simulink model "sl_groundvehicleDynamicsKalman"  (R2025a)
settings: Solver=VariableStepAuto  StartTime=0.0  StopTime=200  FixedStep=0.01  RelTol=1e-5  EnableMultiTasking=on
InitFcn:
  | mdl_robot;
values from neighbouring files (symbols this model uses):
  optimized_waypoints = two_opt_nn_multi_optimisation(cuztomized_wp)    [mdl_robot.m]
undefined symbols (not defined in the file or in its folder): Discrete, robot, Time
libraries: simulink x8, mobileRoboticsLib x5, simulink_extras x2, ctrlSharedLib x1, sharedTrackingLibrary x1
settings Model: Creator=sriramn  LastModifiedBy=login
settings SolverCC: ZeroCrossAlgorithm=Adaptive  AlgebraicLoopSolver=TrustRegion
settings DataIOCC: LimitDataPoints=on  SaveFormat=Array  ReturnWorkspaceOutputs=off
settings OptimizationCC: ReuseModelBlockBuffer=off  LifeSpan=inf
settings DebuggingCC: SolverPrmCheckMsg=warning  UnconnectedInputMsg=warning  UnconnectedOutputMsg=warning  UnconnectedLineMsg=warning  AllowSymbolicDim=off  SFUnexpectedBacktrackingDiag=warning  SFNoUnconditionalDefaultTransitionDiag=warning  SFExecutionAtInitializationDiag=none  ArithmeticOperatorsInVariantConditions=warning
settings HardwareCC: ProdBitPerPointer=32.0  ProdBitPerSizeT=32.0  ProdBitPerPtrDiffT=32.0  ProdLargestAtomicFloat=None  ProdIntDivRoundTo=Undefined  ProdEndianess=Unspecified  ProdWordSize=32.0  ProdHWDeviceType=32-bit Generic
settings ModelReferenceCC: EnableRefExpFcnMdlSchedulingChecks=on  ModelReferenceMinAlgLoopOccurrences=on  PropagateSignalLabelsOutOfModel=off
settings SFSimCC: SimUseLocalCustomCode=off  CustomCodeUndefinedFunction=UseInterfaceOnly
settings RTWCC: RTWUseLocalCustomCode=off  GPUComputeCapability=3.5
settings CodeAppCC: StateflowObjectComments=on
settings GRTTargetCC: TargetLangStandard=C89/C90 (ANSI)
settings ConfigComp: CovMetricSettings=dw  CovSaveCumulativeToWorkspaceVar=on  CovSaveSingleToWorkspaceVar=on  CovExternalEMLEnable=off  CovSFcnEnable=off
settings SimscapeCC: SimscapeLogDataHistory=5000  SimscapeLogDecimation=1  SimscapeNormalizeSystem=off
settings ConfigurationSet: Description=SimMechanics 2G
settings ExplorerConfigSet: InternalSimMechanicsExplorerSettings="<ExplorerConfiguration><canonicalview>planar_xy</canonicalview><AnimationSetting><BasePlaybackSpeed>1.0</BasePlaybackSpeed><PlaybackSpeedFactor>1.0</PlaybackSpeedFactor></AnimationSetting><TilePanel><TileInfo><Tiles Columns=\"1\" Count=\"1\" Rows=\"1\"><Column Left=\"2\" Weight=\"1\"/><Column Left=\"1628\"/><Row Top=\"2\" Weight=\"1\"/><Row Top=\"1072\"/><Tile Height=\"1\" Width=\"1\" X=\"0\" Y=\"0\"/></Tiles></TileInfo><SceneInfo><SceneViewer><BGColor><R>0.60000002384185791</R><G>0.60000002384185791</G><B>0.60000002384185791</B></BGColor><Camera><Position><X>0.22951840878551699</X><Y>0.32651610611526627</Y><Z>-0.27215421354393321</Z></Position><Center><X>-0.15775714411666431</X><Y>-0.15462825985839526</Y><Z>0.065702552916005602</Z></Center><Up><X>-0.56030137557930915</X><Y>0.72817587161684794</Y><Z>0.39474329445726858</Z></Up><Left>-0.21481383955700509</Left><Right>0.21481383955700509</Right><Bottom>-0.27569784609469139</Bottom><Top>0.27569784609469139</Top></Camera></SceneViewer></SceneInfo></TilePanel></ExplorerConfiguration>"

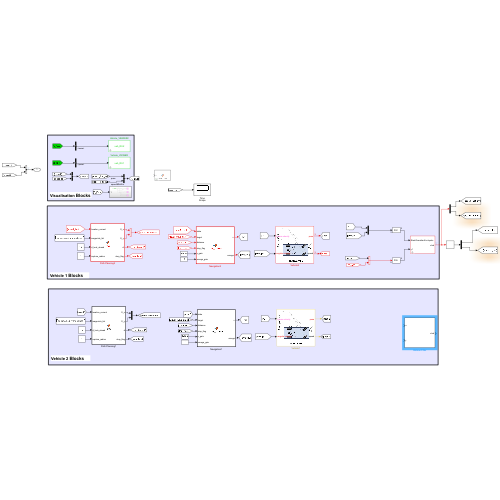
[thumbnail: Simulink's stored preview of the top-level diagram]
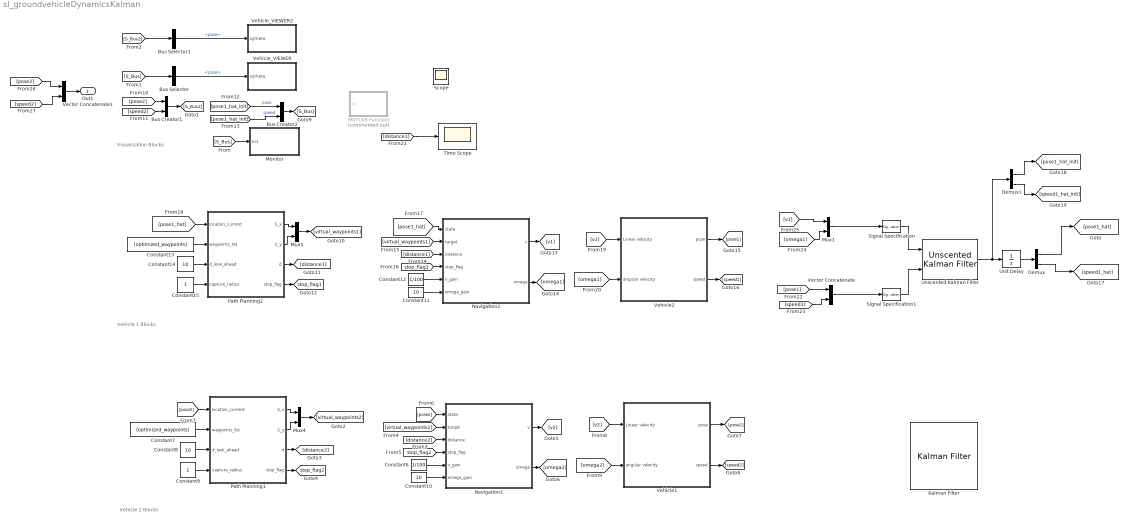
== system sl_groundvehicleDynamicsKalman ==
  note: Visualisation Blocks
  note: Vehicle 1 Blocks
  note: Vehicle 2 Blocks
  Bus Creator1 : BusCreator  Inputs=2
  Bus Creator2 : BusCreator  Inputs=2
  Bus Selector : BusSelector  OutputSignals=pose
  Bus Selector1 : BusSelector  OutputSignals=pose
  Constant{8,10..11,14} (4 alike) : Constant  Value=10
  Constant12 : Constant  Value=1/100
  Constant13 : Constant  Value=[optimized_waypoints]
  Constant15 : Constant
  Constant6 : Constant  Value=1/100
  Constant7 : Constant  Value=[optimized_waypoints]
  Constant9 : Constant
  Demux : Demux  Outputs=2
  Demux1 : Demux  Outputs=2
  Kalman Filter : ctrlSharedLib/Kalman Filter  TimeDomain=Discrete-Time  UseCurrentEstimator=on  ModelSource=LTI State-Space Variable  ModelSourceVariable=ss(0.95,1,1,0,1)  A=0.95  B=1  C=1  D=0  NumberOfStates=1  NumberOfInputs=1  NumberOfOutputs=1  InitialEstimateSource=Dialog  X0=0  P0=10  UseK=off  UseGH=off  NumberOfProcessNoiseInputs=1  G=1  TimeInvariantG=on  H=0  TimeInvariantH=on  Q=0.05  TimeInvariantQ=on  R=1  TimeInvariantR=on  N=0  TimeInvariantN=on  AddInputPort=on  AddEnablePort=off  OutputEstimatedY=off  OutputP=off  Ts=-1
  MATLAB Function : MATLAB Function  Commented=on  TreatAsAtomicUnit=on
  Monitor : Subsystem
  Mux1 : Mux  Inputs=2
  Mux4 : Mux  Inputs=2
  Mux5 : Mux  Inputs=2
  Navigation1 : MATLAB Function  TreatAsAtomicUnit=on
  Navigation2 : MATLAB Function  TreatAsAtomicUnit=on
  Path Planning1 : MATLAB Function  TreatAsAtomicUnit=on
  Path Planning2 : MATLAB Function  TreatAsAtomicUnit=on
  Signal Specification : SignalSpecification  Dimensions=2
  Signal Specification1 : SignalSpecification  Dimensions=6
  Time Scope : Scope
      settings: TimeUnits=Metric (based on Time Span)  ActiveDisplayYMinimum=-32041.582184274124  ActiveDisplayYMaximum=45911.6958514482  YLabel=Amplitude  DataLoggingVariableName=ScopeData3
  Unit Delay : UnitDelay  InitialCondition=[0;0;0;0;0;0]  SampleTime=-1  HasFrameUpgradeWarning=on
  Unscented Kalman Filter : sharedTrackingLibrary/Unscented Kalman Filter  StateTransitionFcn=fState  HasAdditiveProcessNoise=Additive  ProcessNoise=Q  HasTimeVaryingProcessNoise=off  HasStateTransitionFcnExtraArgument=1  InitialState=initial_state  InitialStateCovariance=P0  Alpha=1e-3  Beta=2  Kappa=0  MeasurementFcn1=hMeas  HasMeasurementEnablePort1=off  HasAdditiveMeasurementNoise1=Additive  MeasurementNoise1=R  HasTimeVaryingMeasurementNoise1=off  HasMeasurementFcnExtraArgument1=0  HasMeasurementWrapping1=on  MeasurementFcn2=myMeasurementFcn  HasMeasurementEnablePort2=off  HasAdditiveMeasurementNoise2=Additive  MeasurementNoise2=1  HasTimeVaryingMeasurementNoise2=off  HasMeasurementFcnExtraArgument2=0  HasMeasurementWrapping2=off  MeasurementFcn3=myMeasurementFcn  HasMeasurementEnablePort3=off  HasAdditiveMeasurementNoise3=Additive  MeasurementNoise3=1  HasTimeVaryingMeasurementNoise3=off  HasMeasurementFcnExtraArgument3=0  HasMeasurementWrapping3=off  MeasurementFcn4=myMeasurementFcn  HasMeasurementEnablePort4=off  HasAdditiveMeasurementNoise4=Additive  MeasurementNoise4=1  HasTimeVaryingMeasurementNoise4=off  HasMeasurementFcnExtraArgument4=0  HasMeasurementWrapping4=off  MeasurementFcn5=myMeasurementFcn  HasMeasurementEnablePort5=off  HasAdditiveMeasurementNoise5=Additive  MeasurementNoise5=1  HasTimeVaryingMeasurementNoise5=off  HasMeasurementFcnExtraArgument5=0  HasMeasurementWrapping5=off  EnableMultirate=off  StateTransitionFcnSampleTime=1  MeasurementFcn1SampleTime=1  MeasurementFcn2SampleTime=1  MeasurementFcn3SampleTime=1  MeasurementFcn4SampleTime=1  MeasurementFcn5SampleTime=1  UseCurrentEstimator=on  OutputStateCovariance=off  DataType=double  SampleTime=0.05  NumberOfMeasurements=1
      settings: LibrarySourceBlock=cstblocks/State Estimation/Unscented Kalman Filter
  Vector Concatenate : Concatenate
  Vector Concatenate1 : Concatenate
  Vehicle1 : Subsystem
      mask Display: image('vehicle.jpg');
  Vehicle2 : Subsystem
      mask Display: image('vehicle.jpg');
  Vehicle_VIEWER : Subsystem  mask{wp_mat=optimized_waypoints, veh_ID_num=1, veh_init_xytheta=[robot.X robot.Y robot.Theta], Ts=0.05}
      mask prompts: wp_mat "Waypoint matrix for arena [x_col, y_col] (m)"; veh_ID_num "Vehicle ID number"; veh_init_xytheta "Initial pose [x,y,theta]"; Ts "Sample time for updating animation (secs)"
      mask TypeOptions veh_ID_num: 1 | 2 | 3 | 4
      mask DialogControl Control2 Prompt: Animate simulation of Differential Drive Robot (DDR)
      mask Display: fprintf('veh_ID=%d',veh_ID_num);
  Vehicle_VIEWER2 : Subsystem  mask{wp_mat=optimized_waypoints, veh_ID_num=2, veh_init_xytheta=[robot.X robot.Y robot.Theta], Ts=0.05}
      mask prompts: wp_mat "Waypoint matrix for arena [x_col, y_col] (m)"; veh_ID_num "Vehicle ID number"; veh_init_xytheta "Initial pose [x,y,theta]"; Ts "Sample time for updating animation (secs)"
      mask TypeOptions veh_ID_num: 1 | 2 | 3 | 4
      mask DialogControl Control2 Prompt: Animate simulation of Differential Drive Robot (DDR)
      mask Display: fprintf('veh_ID=%d',veh_ID_num);
  Out1 : Outport
  Scope : Scope
      settings: ActiveDisplayYMinimum=0.07  ActiveDisplayYMaximum=0.09
  tag scope: stop_flag1=global, stop_flag2=global
  wires:
  Constant8/1 -> Path Planning1/3(d_look_ahead)
  Path Planning1/2(S_y) -> Mux4/2
  Constant6/1 -> Navigation1/5(v_gain)
  Constant9/1 -> Path Planning1/4(capture_radius)
  Vehicle1/1(pose) -> [pose2]
  Path Planning1/1(S_x) -> Mux4/1
  Constant7/1 -> Path Planning1/2(waypoints_list)
  Constant10/1 -> Navigation1/6(omega_gain)
  Mux4/1 -> [virtual_waypoints2]
  Path Planning1/3(d) -> [distance2]
  [distance2] -> Navigation1/3(distance)
  [virtual_waypoints2] -> Navigation1/2(target)
  Path Planning1/4(stop_flag) -> [stop_flag2]
  [stop_flag2] -> Navigation1/4(stop_flag)
  Navigation1/1(v) -> [v2]
  Navigation1/2(omega) -> [omega2]
  [pose2] -> Navigation1/1(state)
  [pose2] -> Path Planning1/1(location_current)
  Vehicle1/2(speed) -> [speed2]
  [v2] -> Vehicle1/1(Linear velocity)
  [omega2] -> Vehicle1/2(angular velocity)
  [pose1_hat_init] -> Bus Creator2/1  "pose"
  Bus Creator2/1 -> [S_Bus]
  [pose1_hat_init] -> Bus Creator2/2  "speed"
  Bus Creator1/1 -> [S_Bus2]
  [pose2] -> Bus Creator1/1
  [S_Bus2] -> Bus Selector1/1
  [speed2] -> Bus Creator1/2
  [S_Bus] -> Monitor/1(In1)
  Bus Selector1/1 -> Vehicle_VIEWER2/1(xytheta)  "<pose>"
  Bus Selector/1 -> Vehicle_VIEWER/1(xytheta)  "<pose>"
  [S_Bus] -> Bus Selector/1
  Constant14/1 -> Path Planning2/3(d_look_ahead)
  Navigation2/2(omega) -> [omega1]
  Constant15/1 -> Path Planning2/4(capture_radius)
  Vehicle2/1(pose) -> [pose1]
  Path Planning2/1(S_x) -> Mux5/1
  [stop_flag1] -> Navigation2/4(stop_flag)
  Path Planning2/4(stop_flag) -> [stop_flag1]
  Mux5/1 -> [virtual_waypoints1]
  [pose1_hat] -> Path Planning2/1(location_current)
  Constant11/1 -> Navigation2/6(omega_gain)
  Constant13/1 -> Path Planning2/2(waypoints_list)
  Path Planning2/2(S_y) -> Mux5/2
  [distance1] -> Navigation2/3(distance)
  [v1] -> Vehicle2/1(Linear velocity)
  Constant12/1 -> Navigation2/5(v_gain)
  [omega1] -> Vehicle2/2(angular velocity)
  Path Planning2/3(d) -> [distance1]
  [pose1_hat] -> Navigation2/1(state)
  [virtual_waypoints1] -> Navigation2/2(target)
  Vehicle2/2(speed) -> [speed1]
  Navigation2/1(v) -> [v1]
  [distance1] -> Time Scope/1
  [pose1] -> Vector Concatenate/1
  [speed1] -> Vector Concatenate/2
  Mux1/1 -> Signal Specification/1
  Vector Concatenate/1 -> Signal Specification1/1
  [v1] -> Mux1/1
  [omega1] -> Mux1/2
  Signal Specification/1 -> Unscented Kalman Filter/1
  Signal Specification1/1 -> Unscented Kalman Filter/2
  Demux/1 -> [pose1_hat]
  Demux/2 -> [speed1_hat]
  Unscented Kalman Filter/1 -> Demux1/1, Unit Delay/1
  Unit Delay/1 -> Demux/1
  [pose2] -> Vector Concatenate1/1
  [speed2] -> Vector Concatenate1/2
  Vector Concatenate1/1 -> Out1/1
  Demux1/1 -> [pose1_hat_init]
  Demux1/2 -> [speed1_hat_init]

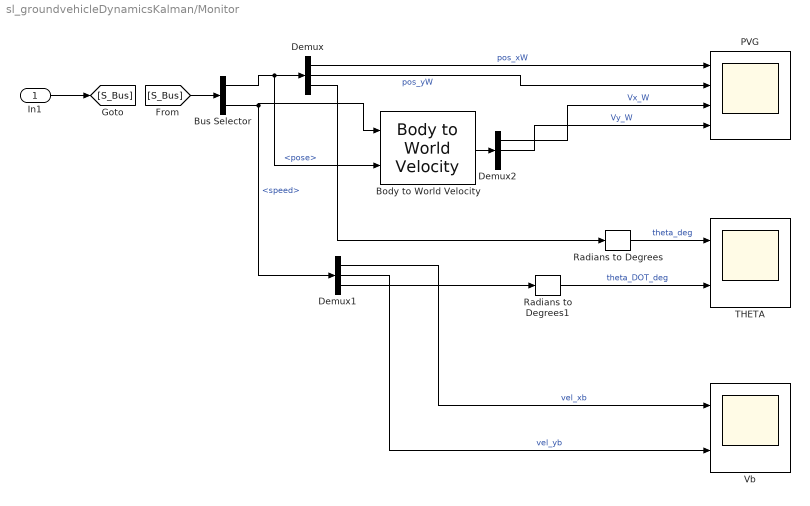
== system sl_groundvehicleDynamicsKalman/Monitor ==
  In1 : Inport
  Body to World Velocity : mobileRoboticsLib/Utilities/Body to World Velocity
      settings: SourceProductName=Mobile Robotics Simulation Toolbox
  Bus Selector : BusSelector  OutputSignals=pose,speed
  Demux : Demux  Outputs=3
  Demux1 : Demux  Outputs=3
  Demux2 : Demux  Outputs=3
  PVG : Scope  NumInputPorts=4
      settings: ActiveDisplayYMinimum=-3.02358  ActiveDisplayYMaximum=27.35477
  Radians to Degrees : simulink_extras/Transformations/Radians to Degrees
  Radians to Degrees1 : simulink_extras/Transformations/Radians to Degrees
  THETA : Scope  NumInputPorts=2
      settings: ActiveDisplayYMinimum=-8.72937  ActiveDisplayYMaximum=60.06611  DataLoggingVariableName=ScopeData2
  Vb : Scope  NumInputPorts=2
      settings: ActiveDisplayYMinimum=0.05577  ActiveDisplayYMaximum=0.8929
  wires:
  In1/1 -> [S_Bus]
  [S_Bus] -> Bus Selector/1
  Demux/1 -> PVG/1  "pos_xW"
  Demux/2 -> PVG/2  "pos_yW"
  Radians to Degrees1/1 -> THETA/2  "theta_DOT_deg"
  Radians to Degrees/1 -> THETA/1  "theta_deg"
  Demux1/3 -> Radians to Degrees1/1
  Demux/3 -> Radians to Degrees/1
  Bus Selector/1 -> Body to World Velocity/2, Demux/1  "<pose>"
  Bus Selector/2 -> Demux1/1, Body to World Velocity/1  "<speed>"
  Body to World Velocity/1 -> Demux2/1
  Demux2/1 -> PVG/3  "Vx_W"
  Demux2/2 -> PVG/4  "Vy_W"
  Demux1/1 -> Vb/1  "vel_xb"
  Demux1/2 -> Vb/2  "vel_yb"

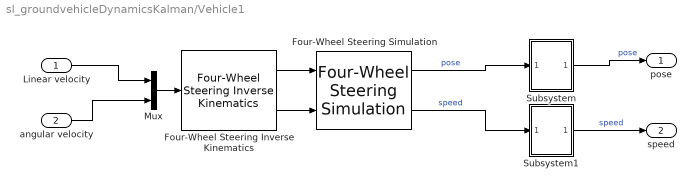
== system sl_groundvehicleDynamicsKalman/Vehicle1 ==
  Linear velocity : Inport
  angular velocity : Inport  Port=2
  Four-Wheel Steering Inverse Kinematics : mobileRoboticsLib/Kinematic Models/Four-Wheel Steering/Four-Wheel Steering Inverse Kinematics  wheelRadius=0.1  frontWheelDist=0.25  rearWheelDist=0.25  ikMode=Front Steering
      settings: SourceProductName=Mobile Robotics Simulation Toolbox
  Four-Wheel Steering Simulation : mobileRoboticsLib/Kinematic Models/Four-Wheel Steering/Four-Wheel Steering Simulation  wheelRadius=0.1  frontWheelDist=0.25  rearWheelDist=0.25  initX=robot.X  initY=robot.Y  initAngle=robot.Theta  Ts=0.05
      settings: SourceProductName=Mobile Robotics Simulation Toolbox
  Mux : Mux  Inputs=2
  Subsystem : Subsystem
  Subsystem1 : Subsystem
  pose : Outport  VectorParamsAs1DForOutWhenUnconnected=off
  speed : Outport  Port=2
  wires:
  angular velocity/1 -> Mux/2
  Linear velocity/1 -> Mux/1
  Mux/1 -> Four-Wheel Steering Inverse Kinematics/1
  Four-Wheel Steering Simulation/1 -> Subsystem/1(In1)  "pose"
  Four-Wheel Steering Simulation/2 -> Subsystem1/1(In1)  "speed"
  Four-Wheel Steering Inverse Kinematics/1 -> Four-Wheel Steering Simulation/1
  Four-Wheel Steering Inverse Kinematics/2 -> Four-Wheel Steering Simulation/2
  Subsystem/1(pose) -> pose/1  "pose"
  Subsystem1/1(speed) -> speed/1  "speed"

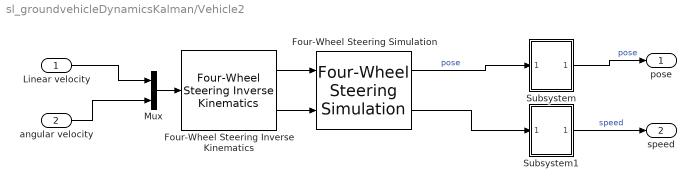
== system sl_groundvehicleDynamicsKalman/Vehicle2 ==
  Linear velocity : Inport
  angular velocity : Inport  Port=2
  Four-Wheel Steering Inverse Kinematics : mobileRoboticsLib/Kinematic Models/Four-Wheel Steering/Four-Wheel Steering Inverse Kinematics  wheelRadius=0.1  frontWheelDist=0.25  rearWheelDist=0.25  ikMode=Front Steering
      settings: SourceProductName=Mobile Robotics Simulation Toolbox
  Four-Wheel Steering Simulation : mobileRoboticsLib/Kinematic Models/Four-Wheel Steering/Four-Wheel Steering Simulation  wheelRadius=0.1  frontWheelDist=0.25  rearWheelDist=0.25  initX=robot.X  initY=robot.Y  initAngle=robot.Theta  Ts=0.05
      settings: SourceProductName=Mobile Robotics Simulation Toolbox
  Mux : Mux  Inputs=2
  Subsystem : Subsystem
  Subsystem1 : Subsystem
  pose : Outport  PortDimensions=3  VectorParamsAs1DForOutWhenUnconnected=off
  speed : Outport  Port=2  PortDimensions=3
  wires:
  angular velocity/1 -> Mux/2
  Linear velocity/1 -> Mux/1
  Mux/1 -> Four-Wheel Steering Inverse Kinematics/1
  Four-Wheel Steering Simulation/1 -> Subsystem/1(In1)  "pose"
  Four-Wheel Steering Inverse Kinematics/1 -> Four-Wheel Steering Simulation/1
  Four-Wheel Steering Inverse Kinematics/2 -> Four-Wheel Steering Simulation/2
  Subsystem/1(pose) -> pose/1  "pose"
  Subsystem1/1(speed) -> speed/1  "speed"
  Four-Wheel Steering Simulation/2 -> Subsystem1/1(In1)

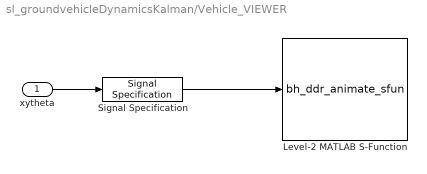
== system sl_groundvehicleDynamicsKalman/Vehicle_VIEWER ==
  xytheta : Inport
  Level-2 MATLAB S-Function : M-S-Function  FunctionName=bh_ddr_animate_sfun  Parameters=Ts, wp_mat, veh_ID_num, veh_init_xytheta
  Signal Specification : SignalSpecification  Dimensions=3
  wires:
  xytheta/1 -> Signal Specification/1
  Signal Specification/1 -> Level-2 MATLAB S-Function/1

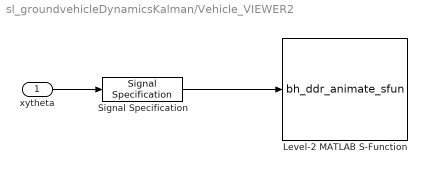
== system sl_groundvehicleDynamicsKalman/Vehicle_VIEWER2 ==
  xytheta : Inport
  Level-2 MATLAB S-Function : M-S-Function  FunctionName=bh_ddr_animate_sfun  Parameters=Ts, wp_mat, veh_ID_num, veh_init_xytheta
  Signal Specification : SignalSpecification  Dimensions=3
  wires:
  xytheta/1 -> Signal Specification/1
  Signal Specification/1 -> Level-2 MATLAB S-Function/1

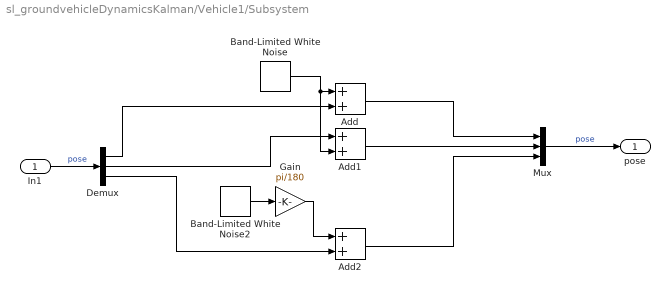
== system sl_groundvehicleDynamicsKalman/Vehicle1/Subsystem ==
  In1 : Inport
  Add : Sum
  Add1 : Sum
  Add2 : Sum
  Band-Limited White Noise : simulink/Sources/Band-Limited White Noise  Cov=[0.001]  Ts=0.1  seed=[23341]
  Band-Limited White Noise2 : simulink/Sources/Band-Limited White Noise  Cov=[0.41]  Ts=0.1  seed=[23341]
  Demux : Demux  Outputs=3
  Gain : Gain  Gain=pi/180
  Mux : Mux  Inputs=3
  pose : Outport
  wires:
  Add1/1 -> Mux/2
  Add2/1 -> Mux/3
  Demux/2 -> Add1/1
  Band-Limited White Noise2/1 -> Gain/1
  Demux/3 -> Add2/2
  Band-Limited White Noise/1 -> Add1/2, Add/1
  In1/1 -> Demux/1  "pose"
  Demux/1 -> Add/2
  Gain/1 -> Add2/1
  Mux/1 -> pose/1  "pose"
  Add/1 -> Mux/1

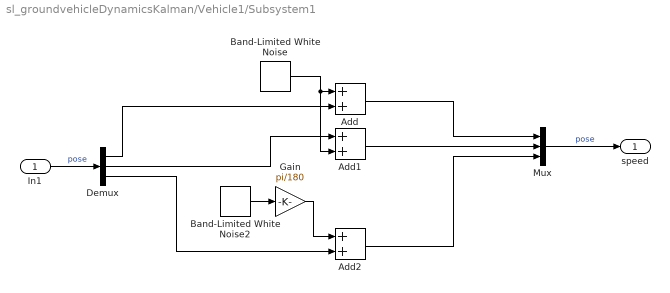
== system sl_groundvehicleDynamicsKalman/Vehicle1/Subsystem1 ==
  In1 : Inport
  Add : Sum
  Add1 : Sum
  Add2 : Sum
  Band-Limited White Noise : simulink/Sources/Band-Limited White Noise  Cov=[0.001]  Ts=0.1  seed=[23341]
  Band-Limited White Noise2 : simulink/Sources/Band-Limited White Noise  Cov=[0.41]  Ts=0.1  seed=[23341]
  Demux : Demux  Outputs=3
  Gain : Gain  Gain=pi/180
  Mux : Mux  Inputs=3
  speed : Outport
  wires:
  Add1/1 -> Mux/2
  Add2/1 -> Mux/3
  Demux/2 -> Add1/1
  Band-Limited White Noise2/1 -> Gain/1
  Demux/3 -> Add2/2
  Band-Limited White Noise/1 -> Add1/2, Add/1
  In1/1 -> Demux/1  "pose"
  Demux/1 -> Add/2
  Gain/1 -> Add2/1
  Mux/1 -> speed/1  "pose"
  Add/1 -> Mux/1

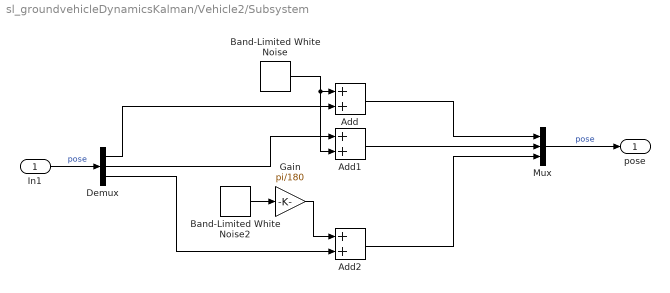
== system sl_groundvehicleDynamicsKalman/Vehicle2/Subsystem ==
  In1 : Inport
  Add : Sum
  Add1 : Sum
  Add2 : Sum
  Band-Limited White Noise : simulink/Sources/Band-Limited White Noise  Cov=[0.001]  Ts=0.1  seed=[23341]
  Band-Limited White Noise2 : simulink/Sources/Band-Limited White Noise  Cov=[0.41]  Ts=0.1  seed=[23341]
  Demux : Demux  Outputs=3
  Gain : Gain  Gain=pi/180
  Mux : Mux  Inputs=3
  pose : Outport
  wires:
  Add1/1 -> Mux/2
  Add2/1 -> Mux/3
  Demux/2 -> Add1/1
  Band-Limited White Noise2/1 -> Gain/1
  Demux/3 -> Add2/2
  Band-Limited White Noise/1 -> Add1/2, Add/1
  In1/1 -> Demux/1  "pose"
  Demux/1 -> Add/2
  Gain/1 -> Add2/1
  Mux/1 -> pose/1  "pose"
  Add/1 -> Mux/1

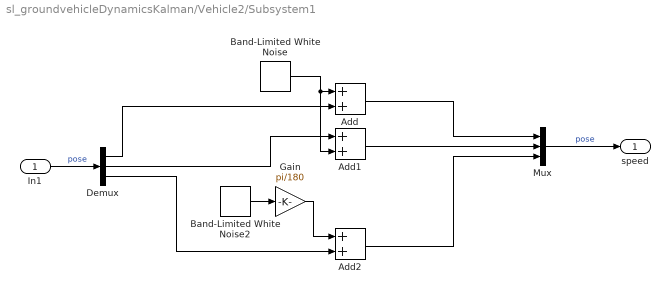
== system sl_groundvehicleDynamicsKalman/Vehicle2/Subsystem1 ==
  In1 : Inport
  Add : Sum
  Add1 : Sum
  Add2 : Sum
  Band-Limited White Noise : simulink/Sources/Band-Limited White Noise  Cov=[0.001]  Ts=0.1  seed=[23341]
  Band-Limited White Noise2 : simulink/Sources/Band-Limited White Noise  Cov=[0.41]  Ts=0.1  seed=[23341]
  Demux : Demux  Outputs=3
  Gain : Gain  Gain=pi/180
  Mux : Mux  Inputs=3
  speed : Outport
  wires:
  Add1/1 -> Mux/2
  Add2/1 -> Mux/3
  Demux/2 -> Add1/1
  Band-Limited White Noise2/1 -> Gain/1
  Demux/3 -> Add2/2
  Band-Limited White Noise/1 -> Add1/2, Add/1
  In1/1 -> Demux/1  "pose"
  Demux/1 -> Add/2
  Gain/1 -> Add2/1
  Mux/1 -> speed/1  "pose"
  Add/1 -> Mux/1

== matlab function sl_groundvehicleDynamicsKalman/MATLAB Function ==
  data: u input
function error_est(u)
    figure(1); clf
    plot(u)
end

== matlab function sl_groundvehicleDynamicsKalman/Navigation1 ==
  data: state input; v output; omega output; target input; distance input; stop_flag input; v_gain input; omega_gain input
function [v, omega] = pure_pursuit(state, target, distance, stop_flag, v_gain, omega_gain)
%PURE_PURSUIT Compute linear and angular velocity using pure pursuit
%   state: [x, y, theta]
%   target: [x_target, y_target]
%   distance: distance to target
%   stop_flag: 0 = move, 1 = stop



% Linear velocity (minimum 0.5 m/s)
v = distance * v_gain;  % Proportional Control
v = max(v, 20);

% Relative position
dx = target(1) - state(1);
dy = target(2) - state(2);

% Line-of-sight angle
gamma = atan2(dy, dx);

% Robot orientation
theta = state(3);

% Pure pursuit angular velocity
omega = omega_gain * angdiff(theta, gamma);
if stop_flag == 1
    v = 0;
    omega = 0;
    return;
end
end

== matlab function sl_groundvehicleDynamicsKalman/Path Planning1 ==
  data: location_current input; S_x output; waypoints_list input; d_look_ahead input; S_y output; d output; stop_flag output; capture_radius input
function [S_x, S_y, d, stop_flag] = RVW(location_current, waypoints_list, d_look_ahead , capture_radius)
    % RVWP computes the Rear-View Waypoint (RVWP) for path following
    
    xd = waypoints_list(:,1);
    yd = waypoints_list(:,2);

    x = location_current(1);
    y = location_current(2);

    % Persistent variable to remember current waypoint index
    persistent n
    if isempty(n)
        n = 1;  % Start from the first waypoint
    end
    stop_flag = 0;
    % Distance to next waypoint
    if n < length(xd)
        stop_flag = 0;
        d = sqrt((x - xd(n+1))^2 + (y - yd(n+1))^2);
        % Distance & angles
        Ru = sqrt((xd(n) - x)^2 + (yd(n) - y)^2);
        theta = atan2(yd(min(n+1,end)) - yd(n), xd(min(n+1,end)) - xd(n));
        theta_u = atan2(y - yd(n), x - xd(n));
        beta = theta - theta_u;
    
        R = Ru * cos(beta);
    
        % Compute RVWP
        S_x = xd(n) + (R + d_look_ahead)*cos(theta);
        S_y = yd(n) + (R + d_look_ahead)*sin(theta);
        if d < capture_radius
            n = n + 1;  % Move to next waypoint
        end
    else
        d = sqrt((x - xd(n))^2 + (y - yd(n))^2);
        S_x = xd(n);
        S_y = yd(n)
        if d < 1
            stop_flag = 1;
        end
    end
end

== matlab function sl_groundvehicleDynamicsKalman/Navigation2 ==
  data: state input; v output; omega output; target input; distance input; stop_flag input; v_gain input; omega_gain input
function [v, omega] = pure_pursuit(state, target, distance, stop_flag, v_gain, omega_gain)
%PURE_PURSUIT Compute linear and angular velocity using pure pursuit
%   state: [x, y, theta]
%   target: [x_target, y_target]
%   distance: distance to target
%   stop_flag: 0 = move, 1 = stop



% Linear velocity (minimum 0.5 m/s)
v = distance * v_gain;  % Proportional Control
v = max(v, 20);

% Relative position
dx = target(1) - state(1);
dy = target(2) - state(2);

% Line-of-sight angle
gamma = atan2(dy, dx);

% Robot orientation
theta = state(3);

% Pure pursuit angular velocity
omega = omega_gain * angdiff(theta, gamma);
if stop_flag == 1
    v = 0;
    omega = 0;
    return;
end
end

== matlab function sl_groundvehicleDynamicsKalman/Path Planning2 ==
  data: location_current input; S_x output; waypoints_list input; d_look_ahead input; S_y output; d output; stop_flag output; capture_radius input
function [S_x, S_y, d, stop_flag] = RVW(location_current, waypoints_list, d_look_ahead , capture_radius)
    % RVWP computes the Rear-View Waypoint (RVWP) for path following
    
    xd = waypoints_list(:,1);
    yd = waypoints_list(:,2);

    x = location_current(1);
    y = location_current(2);

    % Persistent variable to remember current waypoint index
    persistent n
    if isempty(n)
        n = 1;  % Start from the first waypoint
    end
    stop_flag = 0;
    % Distance to next waypoint
    if n < length(xd)
        stop_flag = 0;
        d = sqrt((x - xd(n+1))^2 + (y - yd(n+1))^2);
        % Distance & angles
        Ru = sqrt((xd(n) - x)^2 + (yd(n) - y)^2);
        theta = atan2(yd(min(n+1,end)) - yd(n), xd(min(n+1,end)) - xd(n));
        theta_u = atan2(y - yd(n), x - xd(n));
        beta = theta - theta_u;
    
        R = Ru * cos(beta);
    
        % Compute RVWP
        S_x = xd(n) + (R + d_look_ahead)*cos(theta);
        S_y = yd(n) + (R + d_look_ahead)*sin(theta);
        if d < capture_radius
            n = n + 1;  % Move to next waypoint
        end
    else
        d = sqrt((x - xd(n))^2 + (y - yd(n))^2);
        S_x = xd(n);
        S_y = yd(n)
        if d < 1
            stop_flag = 1;
        end
    end
end
